simulink model "part12"  (R2017b)
settings: Solver=VariableStepAuto  StartTime=0.0  StopTime=50  RelTol=1e-3
settings Model: Creator=admin  LastModifiedBy=admin

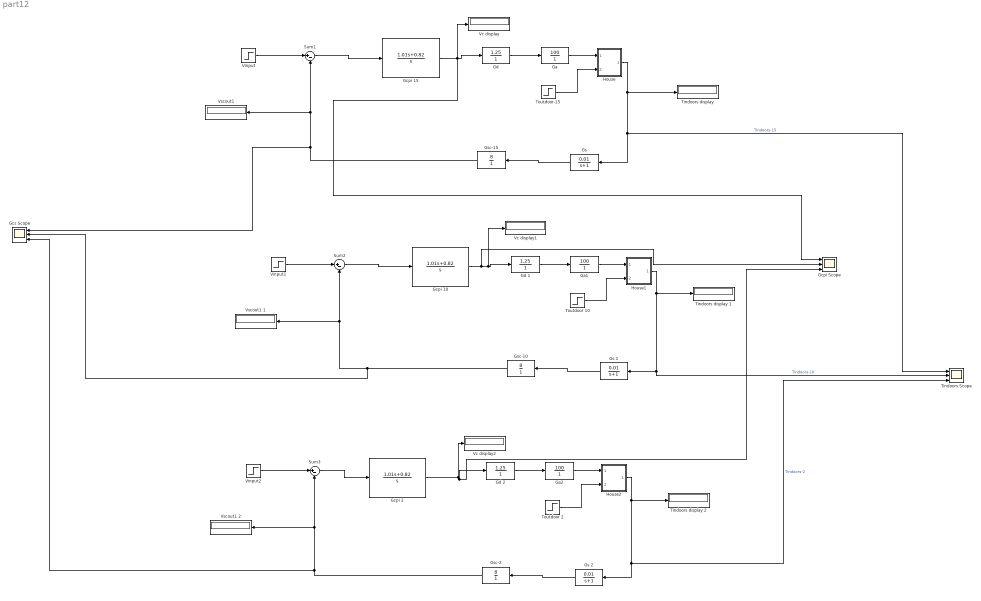
== system part12 ==
  Ga : TransferFcn  Numerator=[100]  Denominator=[1 ]
  Ga1 : TransferFcn  Numerator=[100]  Denominator=[1 ]
  Ga2 : TransferFcn  Numerator=[100]  Denominator=[1 ]
  Gcpi 10 : TransferFcn  Numerator=[1.01 0.82]  Denominator=[1 0]
  "Gcpi 15 " : TransferFcn  Numerator=[1.01 0.82]  Denominator=[1 0]
  Gcpi 2 : TransferFcn  Numerator=[1.01 0.82]  Denominator=[1 0]
  Gcpi Scope : Scope  NumInputPorts=3
  Gcs Scope : Scope  NumInputPorts=3
  "Gd " : TransferFcn  Numerator=[1.25]  Denominator=[1 ]
  Gd 1 : TransferFcn  Numerator=[1.25]  Denominator=[1 ]
  Gd 2 : TransferFcn  Numerator=[1.25]  Denominator=[1 ]
  "Gs " : TransferFcn  Numerator=[0.01]  Denominator=[1 1]
  Gs 1 : TransferFcn  Numerator=[0.01]  Denominator=[1 1]
  Gs 2 : TransferFcn  Numerator=[0.01]  Denominator=[1 1]
  Gsc-10 : TransferFcn  Numerator=[8]  Denominator=[1 ]
  Gsc-15 : TransferFcn  Numerator=[8]  Denominator=[1 ]
  Gsc-2 : TransferFcn  Numerator=[8]  Denominator=[1 ]
  House : Subsystem
      mask Display: image(fullfile(matlabroot,'toolbox','simulink','simdemos','simgeneral','images','HouseHeatHousePix.svg'))
  House1 : Subsystem
      mask Display: image(fullfile(matlabroot,'toolbox','simulink','simdemos','simgeneral','images','HouseHeatHousePix.svg'))
  House2 : Subsystem
      mask Display: image(fullfile(matlabroot,'toolbox','simulink','simdemos','simgeneral','images','HouseHeatHousePix.svg'))
  Sum1 : Sum  Inputs=|+-
  Sum2 : Sum  Inputs=|+-
  Sum3 : Sum  Inputs=|+-
  "Tindoors Scope " : Scope  NumInputPorts=3
  "Tindoors display " : Display
  Tindoors display 1 : Display
  Tindoors display 2 : Display
  Toutdoor 10 : Step  Time=0  After=10  SampleTime=0
  Toutdoor 2 : Step  Time=0  After=2  SampleTime=0
  "Toutdoor-15 " : Step  Time=0  After=15  SampleTime=0
  Vc display : Display
  Vc display1 : Display
  Vc display2 : Display
  Vinput : Step  Time=0  After=2.06  SampleTime=0
  Vinput1 : Step  Time=0  After=2.06  SampleTime=0
  Vinput2 : Step  Time=0  After=2.06  SampleTime=0
  "Vscout1 " : Display
  Vscout1 1 : Display
  Vscout1 2 : Display
  wires:
  "Toutdoor-15 "/1 -> House/2(Outdoor Temp Tout)
  "Gs "/1 -> Gsc-15/1
  House/1(Room Temp Troom) -> "Tindoors display "/1, "Tindoors Scope "/1, "Gs "/1  "Tindoors-15"
  "Gcpi 15 "/1 -> Gcpi Scope/1, Vc display/1, "Gd "/1
  Gsc-15/1 -> Gcs Scope/1, "Vscout1 "/1, Sum1/2
  Sum1/1 -> "Gcpi 15 "/1
  "Gd "/1 -> Ga/1
  Vinput/1 -> Sum1/1
  Ga/1 -> House/1(Heater QDot In)
  Ga1/1 -> House1/1(Heater QDot In)
  Gd 1/1 -> Ga1/1
  Vinput1/1 -> Sum2/1
  Sum2/1 -> Gcpi 10/1
  Gsc-10/1 -> Gcs Scope/2, Vscout1 1/1, Sum2/2
  House1/1(Room Temp Troom) -> Tindoors display 1/1, "Tindoors Scope "/2, Gs 1/1  "Tindoors-10"
  Gs 1/1 -> Gsc-10/1
  Gcpi 10/1 -> Gcpi Scope/2, Vc display1/1, Gd 1/1
  Toutdoor 10/1 -> House1/2(Outdoor Temp Tout)
  Ga2/1 -> House2/1(Heater QDot In)
  Gd 2/1 -> Ga2/1
  Vinput2/1 -> Sum3/1
  Sum3/1 -> Gcpi 2/1
  Gsc-2/1 -> Gcs Scope/3, Vscout1 2/1, Sum3/2
  House2/1(Room Temp Troom) -> Tindoors display 2/1, "Tindoors Scope "/3, Gs 2/1  "Tindoors-2"
  Gs 2/1 -> Gsc-2/1
  Gcpi 2/1 -> Vc display2/1, Gcpi Scope/3, Gd 2/1
  Toutdoor 2/1 -> House2/2(Outdoor Temp Tout)

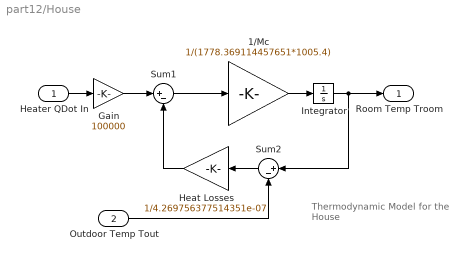
== system part12/House ==
  note: Thermodynamic Model
      | for the House
  Heater QDot In : Inport
  Outdoor Temp Tout : Inport  Port=2
  1/Mc : Gain  Gain=1/(1778.369114457651*1005.4)  SaturateOnIntegerOverflow=on  OutDataTypeStr=Inherit: Same as input  ParamDataTypeStr=Inherit: Same as input
  Gain : Gain  Gain=100000
  Heat Losses : Gain  Gain=1/4.269756377514351e-07  SaturateOnIntegerOverflow=on  OutDataTypeStr=Inherit: Same as input  ParamDataTypeStr=Inherit: Same as input
  Integrator : Integrator  InitialCondition=20
  Sum1 : Sum  Inputs=|+-  SaturateOnIntegerOverflow=on  InputSameDT=on  OutDataTypeStr=Inherit: Same as first input
  Sum2 : Sum  Inputs=|+-  SaturateOnIntegerOverflow=on  InputSameDT=on  OutDataTypeStr=Inherit: Same as first input
  Room Temp Troom : Outport  InitialOutput=0
  wires:
  Outdoor Temp Tout/1 -> Sum2/2
  Heater QDot In/1 -> Gain/1
  Sum1/1 -> 1/Mc/1
  Sum2/1 -> Heat Losses/1
  Heat Losses/1 -> Sum1/2
  1/Mc/1 -> Integrator/1
  Integrator/1 -> Sum2/1, Room Temp Troom/1
  Gain/1 -> Sum1/1

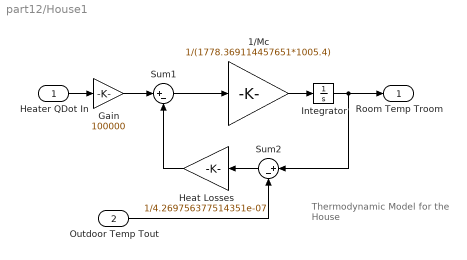
== system part12/House1 ==
  note: Thermodynamic Model
      | for the House
  Heater QDot In : Inport
  Outdoor Temp Tout : Inport  Port=2
  1/Mc : Gain  Gain=1/(1778.369114457651*1005.4)  SaturateOnIntegerOverflow=on  OutDataTypeStr=Inherit: Same as input  ParamDataTypeStr=Inherit: Same as input
  Gain : Gain  Gain=100000
  Heat Losses : Gain  Gain=1/4.269756377514351e-07  SaturateOnIntegerOverflow=on  OutDataTypeStr=Inherit: Same as input  ParamDataTypeStr=Inherit: Same as input
  Integrator : Integrator  InitialCondition=20
  Sum1 : Sum  Inputs=|+-  SaturateOnIntegerOverflow=on  InputSameDT=on  OutDataTypeStr=Inherit: Same as first input
  Sum2 : Sum  Inputs=|+-  SaturateOnIntegerOverflow=on  InputSameDT=on  OutDataTypeStr=Inherit: Same as first input
  Room Temp Troom : Outport  InitialOutput=0
  wires:
  Outdoor Temp Tout/1 -> Sum2/2
  Heater QDot In/1 -> Gain/1
  Sum1/1 -> 1/Mc/1
  Sum2/1 -> Heat Losses/1
  Heat Losses/1 -> Sum1/2
  1/Mc/1 -> Integrator/1
  Integrator/1 -> Sum2/1, Room Temp Troom/1
  Gain/1 -> Sum1/1

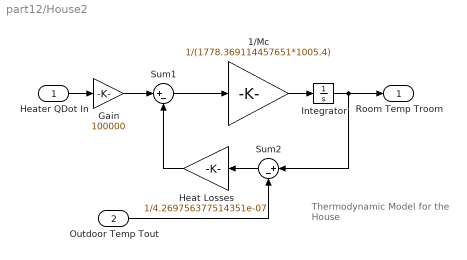
== system part12/House2 ==
  note: Thermodynamic Model
      | for the House
  Heater QDot In : Inport
  Outdoor Temp Tout : Inport  Port=2
  1/Mc : Gain  Gain=1/(1778.369114457651*1005.4)  SaturateOnIntegerOverflow=on  OutDataTypeStr=Inherit: Same as input  ParamDataTypeStr=Inherit: Same as input
  Gain : Gain  Gain=100000
  Heat Losses : Gain  Gain=1/4.269756377514351e-07  SaturateOnIntegerOverflow=on  OutDataTypeStr=Inherit: Same as input  ParamDataTypeStr=Inherit: Same as input
  Integrator : Integrator  InitialCondition=20
  Sum1 : Sum  Inputs=|+-  SaturateOnIntegerOverflow=on  InputSameDT=on  OutDataTypeStr=Inherit: Same as first input
  Sum2 : Sum  Inputs=|+-  SaturateOnIntegerOverflow=on  InputSameDT=on  OutDataTypeStr=Inherit: Same as first input
  Room Temp Troom : Outport  InitialOutput=0
  wires:
  Outdoor Temp Tout/1 -> Sum2/2
  Heater QDot In/1 -> Gain/1
  Sum1/1 -> 1/Mc/1
  Sum2/1 -> Heat Losses/1
  Heat Losses/1 -> Sum1/2
  1/Mc/1 -> Integrator/1
  Integrator/1 -> Sum2/1, Room Temp Troom/1
  Gain/1 -> Sum1/1
